simulink model "power_dashboard"  (R2022b)
settings: Solver=FixedStepAuto  StartTime=0.0  StopTime=200  FixedStep=0.1  RelTol=1e-3
settings Model: PacingRate=3  Creator=Brigosha_Guest  LastModifiedBy=Brigosha_Guest

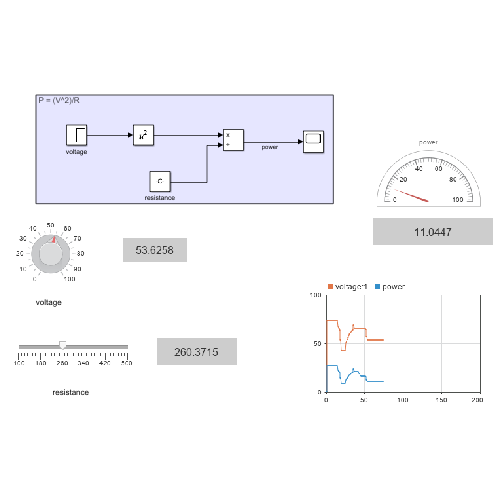
[thumbnail: Simulink's stored preview of the top-level diagram]
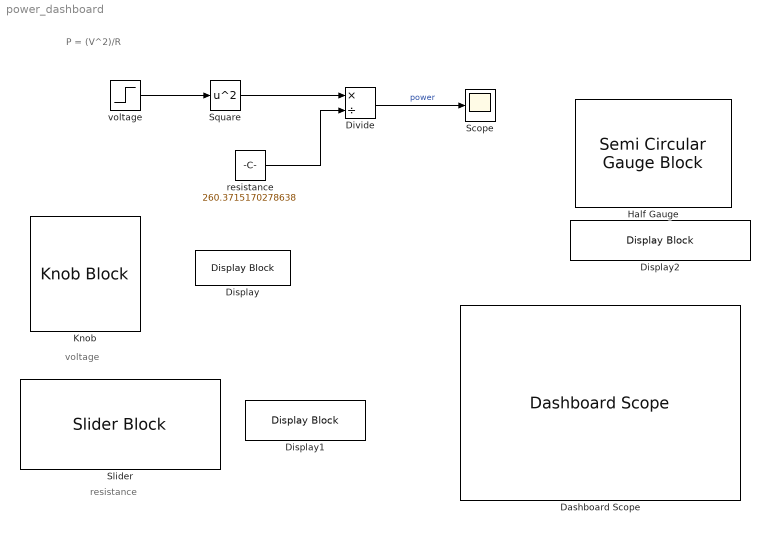
== system power_dashboard ==
  note: P = (V^2)/R
  note: voltage
  note: resistance
  Dashboard Scope : DashboardScope  Ymin=0  Ymax=100  ScaleAtStop=off  UpdateMode=Scroll
  Display : DisplayBlock  LabelPosition=Hide  Transparency=1
  Display1 : DisplayBlock  LabelPosition=Hide  Transparency=1
  Display2 : DisplayBlock  LabelPosition=Hide  Transparency=1
  Divide : Product  Inputs=*/
  Half Gauge : SemiCircularGaugeBlock
  Knob : KnobBlock  LabelPosition=Hide
  Scope : Scope
  Slider : SliderBlock  LabelPosition=Hide  ScaleMin=100  ScaleMax=500
  Square : Math  Operator=square
  resistance : Constant  Value=260.3715170278638
  voltage : Step  After=53.62579345703125  SampleTime=0
  wires:
  voltage/1 -> Square/1
  resistance/1 -> Divide/2
  Divide/1 -> Scope/1  "power"
  Square/1 -> Divide/1
